simulink model "Driver_Glider"  (R2018a)
settings: Solver=ode45  StartTime=0.0  StopTime=TimeUS06  MaxStep=.1  RelTol=1e-3  EnableMultiTasking=on
PostLoadFcn:
  | GliderDir = pwd;
  | 
  | cd ..\;
  | SimulinkDir = pwd;
  | addpath(SimulinkDir);
  | 
  | cd(GliderDir);
model workspace (MAT data in the model file):
  DrCycles : struct (value not decoded)
  DriverPic = [255 255 255 255 255 255 255 255 255 255 255 255 ... (1049040 elements, 940x372x3)]
  TimeHWFET = 765
  TimeUDDS = 1372
  TimeUS06 = 596
  VehiclePic = [252 252 252 252 252 252 252 252 252 252 252 252 ... (1047540 elements, 316x1105x3)]
  aeroDragCoeff = 0.38
  airDensity = 1.23
  frontArea = 2.1
  gravity = 9.81
  inclinationAngle = 0
  inertialMassVeh = 2392
  massVeh = 2300
  rollingResistCoeff = 0.01
libraries: simulink x1, Driver_Glider_Library x1
(part 2 of 2)

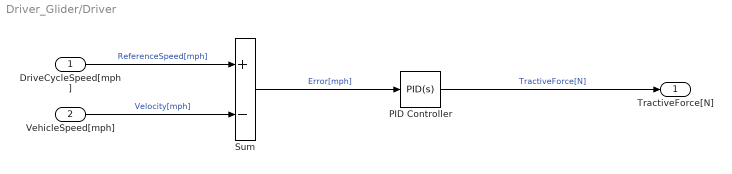
== system Driver_Glider/Driver ==
  DriveCycleSpeed[mph] : Inport
  VehicleSpeed[mph] : Inport  Port=2
  PID Controller : simulink/Continuous/PID Controller  Controller=PID  TimeDomain=Continuous-time  SampleTime=-1  IntegratorMethod=Forward Euler  FilterMethod=Forward Euler  Form=Parallel  UseFilter=on  ControllerParametersSource=internal  P=7500  I=1  D=0  N=100  InitialConditionSource=internal  InitialConditionForIntegrator=0  InitialConditionForFilter=0  ExternalReset=none  LimitOutput=off  UpperSaturationLimit=inf  LowerSaturationLimit=-inf  LinearizeAsGain=on  AntiWindupMode=none  Kb=1  TrackingMode=off  Kt=1  PParamMin=[]  PParamMax=[]  IParamMin=[]  IParamMax=[]  DParamMin=[]  DParamMax=[]  NParamMin=[]  NParamMax=[]  KbParamMin=[]  KbParamMax=[]  KtParamMin=[]  KtParamMax=[]  POutMin=[]  POutMax=[]  IOutMin=[]  IOutMax=[]  DOutMin=[]  DOutMax=[]  NOutMin=[]  NOutMax=[]  KbOutMin=[]  KbOutMax=[]  KtOutMin=[]  KtOutMax=[]  IntegratorOutMin=[]  IntegratorOutMax=[]  FilterOutMin=[]  FilterOutMax=[]  SumOutMin=[]  SumOutMax=[]  SumI1OutMin=[]  SumI1OutMax=[]  SumI2OutMin=[]  SumI2OutMax=[]  SumI3OutMin=[]  SumI3OutMax=[]  SumDOutMin=[]  SumDOutMax=[]  SaturationOutMin=[]  SaturationOutMax=[]  IntegratorContinuousStateAttributes=''  IntegratorStateMustResolveToSignalObject=off  IntegratorRTWStateStorageClass=Auto  FilterContinuousStateAttributes=''  FilterStateMustResolveToSignalObject=off  FilterRTWStateStorageClass=Auto  DifferentiatorICPrevScaledInput=0  DifferentiatorOutMin=[]  DifferentiatorOutMax=[]  InitialConditionSetting=State (most efficient)  FilterDiffOutCoefMin=[]  FilterDiffOutCoefMax=[]  SumDenOutMin=[]  SumDenOutMax=[]  SumNumOutMin=[]  SumNumOutMax=[]  ReciprocalOutMin=[]  ReciprocalOutMax=[]  DivideOutMin=[]  DivideOutMax=[]  TunerSelectOption=Transfer Function Based (PID Tuner App)
  Sum : Sum  Inputs=+-
  TractiveForce[N] : Outport
  wires:
  DriveCycleSpeed[mph]/1 -> Sum/1  "ReferenceSpeed[mph]"
  Sum/1 -> PID Controller/1  "Error[mph]"
  VehicleSpeed[mph]/1 -> Sum/2  "Velocity[mph]"
  PID Controller/1 -> TractiveForce[N]/1  "TractiveForce[N]"
